simulink model "Controlador1_Simulink"  (R2019a)
settings: Solver=VariableStepAuto  StartTime=0.0  StopTime=10  RelTol=1e-3
values from neighbouring files (symbols this model uses):
  A = [0 1 0 ; 0 0 1 ; 0 -2 -3]    [controlador_espaco_de_estados_1.m]    (also in controlador_espaco_de_estados_2.m; controlador_espaco_de_estados_3.m; controlador_espaco_de_estados_4.m = [0 1 ; 1 0]; controlador_espaco_de_estados_5.m = [0 1 0 ; 0 0 1 ; 0 -200 -30])
  B = [0 ; 0 ; 1]    [controlador_espaco_de_estados_1.m]    (also in controlador_espaco_de_estados_2.m; controlador_espaco_de_estados_3.m; controlador_espaco_de_estados_4.m = [0 ; 1]; controlador_espaco_de_estados_5.m)
  K = place(A, B, desired_poles)    [controlador_espaco_de_estados_1.m]    (also in controlador_espaco_de_estados_2.m = place(A, B, [s1, s2, s3]); controlador_espaco_de_estados_3.m = place(A, B, [s1 s2 s3]); controlador_espaco_de_estados_4.m = [0 1] * inv(M) * phi; controlador_espaco_de_estados_5.m = [2600 352 30])
settings Model: Creator=rcard  LastModifiedBy=rcard

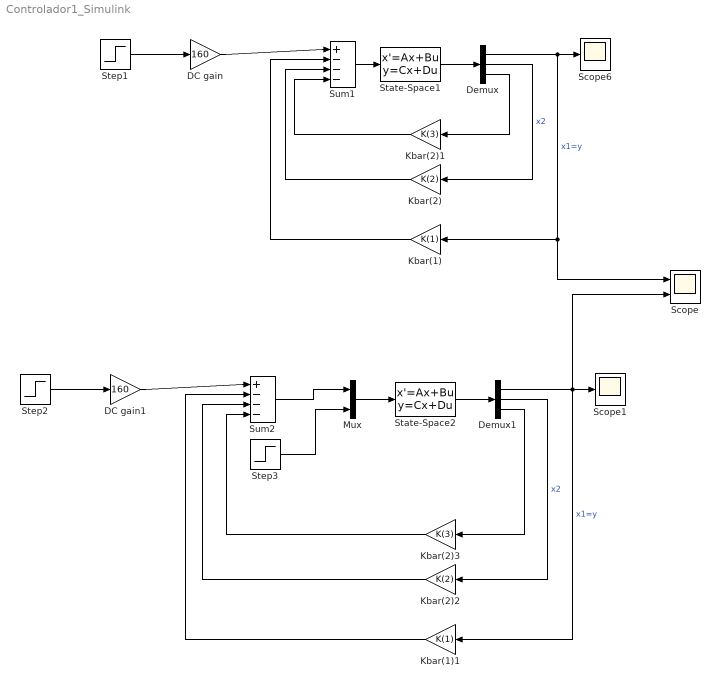
== system Controlador1_Simulink ==
  DC gain : Gain  Gain=160
  DC gain1 : Gain  Gain=160
  Demux : Demux  Outputs=3
  Demux1 : Demux  Outputs=3
  Kbar(1) : Gain  Gain=K(1)
  Kbar(1)1 : Gain  Gain=K(1)
  Kbar(2) : Gain  Gain=K(2)
  Kbar(2)1 : Gain  Gain=K(3)
  Kbar(2)2 : Gain  Gain=K(2)
  Kbar(2)3 : Gain  Gain=K(3)
  Mux : Mux  Inputs=2
  Scope : Scope  NumInputPorts=2
  Scope1 : Scope
  Scope6 : Scope
  State-Space1 : StateSpace  A=A  B=B  C=eye(3)  D=zeros(3,1)  InitialCondition=[0 0 0]
  State-Space2 : StateSpace  A=A  B=[B -B]  C=eye(3)  D=zeros(3,2)  InitialCondition=[0 0 0]
  Step1 : Step  Time=0  SampleTime=1/20000
  Step2 : Step  Time=0  SampleTime=1/20000
  Step3 : Step  Time=5  After=5  SampleTime=1/20000
  Sum1 : Sum  Inputs=|+---
  Sum2 : Sum  Inputs=|+---
  wires:
  Sum1/1 -> State-Space1/1
  Step1/1 -> DC gain/1
  State-Space1/1 -> Demux/1
  Demux/1 -> Scope/1, Kbar(1)/1, Scope6/1  "x1=y"
  Demux/2 -> Kbar(2)/1  "x2"
  Kbar(2)/1 -> Sum1/3
  Kbar(1)/1 -> Sum1/2
  Demux/3 -> Kbar(2)1/1
  Kbar(2)1/1 -> Sum1/4
  DC gain/1 -> Sum1/1
  DC gain1/1 -> Sum2/1
  Step2/1 -> DC gain1/1
  Kbar(2)2/1 -> Sum2/3
  State-Space2/1 -> Demux1/1
  Demux1/2 -> Kbar(2)2/1  "x2"
  Kbar(2)3/1 -> Sum2/4
  Demux1/3 -> Kbar(2)3/1
  Kbar(1)1/1 -> Sum2/2
  Demux1/1 -> Scope/2, Kbar(1)1/1, Scope1/1  "x1=y"
  Mux/1 -> State-Space2/1
  Sum2/1 -> Mux/1
  Step3/1 -> Mux/2
